simulink library "sf_atomic_sensor_lib"  (Simulink 7.6)
settings: Solver=ode45  StartTime=0.0  StopTime=10.0  RelTol=1e-3
undefined symbols (not defined in the file or in its folder): HIGH, LOW
settings Model: Creator=The MathWorks Inc.

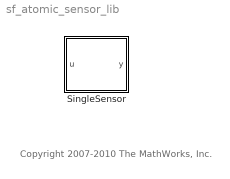
== system sf_atomic_sensor_lib ==
  note: Copyright 2007-2010 The MathWorks, Inc.
  SingleSensor : Stateflow chart  TreatAsAtomicUnit=on

== stateflow chart SingleSensor ==
  state yn = inFailed [function]
    (default) -> (junction 9) : {yn = in(Fail);}
  state OK
    en, du: y = u;
  state Fail
    en, du: y = 0;
  state FailOnce
  state yn = readingOK [function]
    (default) -> (junction 8) : {yn = (u > LOW && u < HIGH);}
  OK -> FailOnce : [!readingOK()]
  FailOnce -> OK [order 2] : [readingOK()]
  FailOnce -> Fail [order 1] : [after(0.5,sec)]
  (default) -> OK
  data: yn function_output double; yn function_output double; u input double; y output double; HIGH parameter double; LOW parameter double
